simulink model "full_diffdrive_ctrl_sim_and_exp_with_arduino"  (R2020a)
settings: Solver=ode3  StartTime=0.0  StopTime=20  FixedStep=0.01  RelTol=1e-3  EnableMultiTasking=on
libraries: xpcobsoletelib x11, simulink x9, arduinolib x4, xpcutilitieslib x3, xpcrtudplib x2, slrtlib x1
(part 1 of 2)
settings Model: SILPILModeSetting=veronly  ExtModeTrigDuration=2  Creator=Boreth  LastModifiedBy=Boreth
settings DataIOCC: ReturnWorkspaceOutputs=off
settings OptimizationCC: EnhancedBackFolding=on  PassReuseOutputArgsAs=Individual arguments  MaxStackSize=64  OptimizeBlockOrder=speed  DifferentSizesBufferReuse=on  OptimizationCustomize=off  EfficientTunableParamExpr=on
settings DebuggingCC: InheritedTsInSrcMsg=none  ParameterTunabilityLossMsg=error  ArithmeticOperatorsInVariantConditions=warning
settings HardwareCC: ProdBitPerPointer=32  ProdBitPerSizeT=32  ProdBitPerPtrDiffT=32  ProdLargestAtomicInteger=Long  ProdLargestAtomicFloat=Double  ProdWordSize=32  ProdHWDeviceType=ARM Compatible->ARM Cortex
settings SFSimCC: MATLABDynamicMemAlloc=off  CustomCodeUndefinedFunction=UseInterfaceOnly
settings RTWCC: SystemTargetFile=ert.tlc  HardwareBoard=Arduino Due  TLCOptions=-aInlineSetEventsForThisBaseRateFcn=TLC_FALSE -aSuppressMultiTaskScheduler=TLC_FALSE -aRateBasedStepFcn=1  TemplateMakefile=ert_default_tmf  GenerateReport=on  Toolchain=Arduino ARM  BuildConfiguration=Faster Runs  IncludeHyperlinkInReport=on  LaunchReport=on  GenerateTraceInfo=on  GenerateTraceReport=on  GenerateTraceReportSl=on  GenerateTraceReportSf=on  GenerateTraceReportEml=on
settings CodeAppCC: ForceParamTrailComments=on  IgnoreCustomStorageClasses=off  OperatorAnnotations=on  SimulinkDataObjDesc=on  SFDataObjDesc=on  InsertBlockDesc=on
settings ERTTargetCC: SupportContinuousTime=on  SupportVariableSizeSignals=on  ExtModeStaticAllocSize=24576

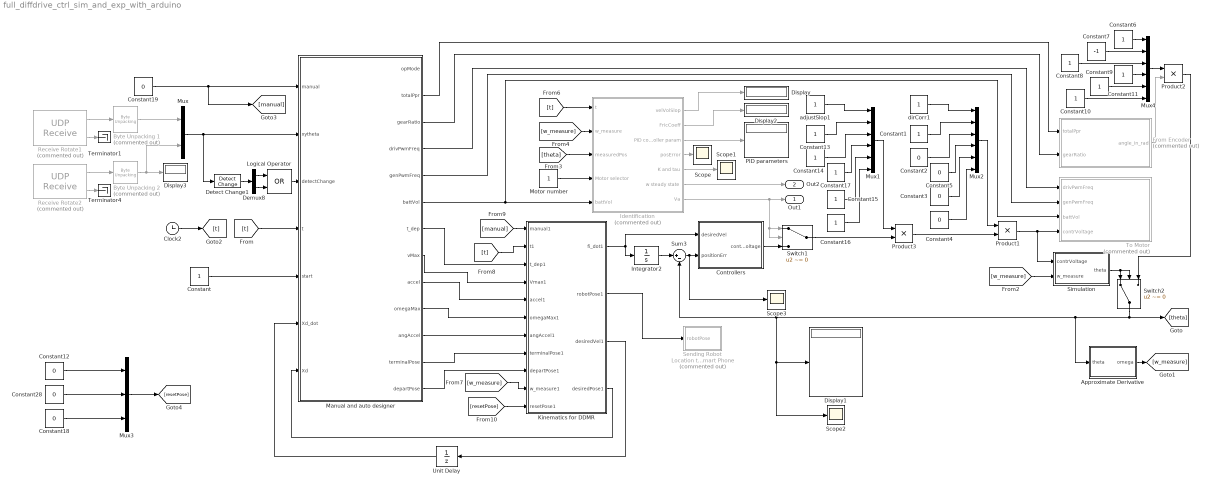
== system full_diffdrive_ctrl_sim_and_exp_with_arduino ==
  Approximate Derivative : Subsystem
  Byte Unpacking 1 : xpcutilitieslib/Byte Unpacking   Commented=on  MaskUnpackedDataTypes={'double'}  MaskUnpackedDataSizes={[1]}  MaskAlignment=1
      settings: SourceProductBaseCode=XP
  Byte Unpacking 2 : xpcutilitieslib/Byte Unpacking   Commented=on  MaskUnpackedDataTypes={'double'}  MaskUnpackedDataSizes={[1]}  MaskAlignment=1
      settings: SourceProductBaseCode=XP
  Clock2 : Clock
  Constant{,1,6,8..11,13..17} (12 alike) : Constant
  Constant{2..5,12,18..19,28} (8 alike) : Constant  Value=0
  Constant7 : Constant  Value=-1
  Controllers : Subsystem
  Demux8 : Demux  Outputs=2
  Detect Change1 : simulink/Logic and Bit Operations/Detect Change  vinit=0  OutDataTypeStr=boolean
  Display{,1..3} (4 alike) : Display
  From Encoder : Subsystem  Commented=on
  Identification : Subsystem  Commented=on
  Integrator2 : Integrator  InitialCondition=zeros(6,1)
  Kinematics for DDMR : Subsystem
  Logical Operator : Logic  Operator=OR  AllPortsSameDT=off  OutDataTypeStr=boolean
  Manual and auto designer : Stateflow chart  TreatAsAtomicUnit=on
  Motor number : Constant
  Mux : Mux  Inputs=2
  Mux1 : Mux  Inputs=6
  Mux2 : Mux  Inputs=6
  Mux3 : Mux  Inputs=3
  Mux4 : Mux  Inputs=6
  PID parameters : Display
  Product1 : Product
  Product2 : Product
  Product3 : Product
  Receive Rotate1 : xpcrtudplib/UDP Receive  Commented=on  ipAddressVal=Use host-target connection  localPort=2501  rcvWidth=8  rcvFmAny=off  fmAddress=192.168.88.233  rcvMulticast=off  multicastAddress={}  maxUDPQueue=8  sampleTime=-1
  Receive Rotate2 : xpcrtudplib/UDP Receive  Commented=on  ipAddressVal=Use host-target connection  localPort=2502  rcvWidth=8  rcvFmAny=off  fmAddress=192.168.88.233  rcvMulticast=off  multicastAddress={}  maxUDPQueue=8  sampleTime=-1
  Scope{,1..3} (4 alike) : Scope
  Sending Robot Location to Smart Phone : Subsystem  Commented=on
  Simulation : Subsystem
  Sum3 : Sum  Inputs=|+-
  Switch1 : Switch  Criteria=u2 ~= 0
  Switch2 : Switch  Criteria=u2 ~= 0
  Terminator1 : Terminator
  Terminator4 : Terminator
  To Motor : Subsystem  Commented=on
  Unit Delay : UnitDelay  InitialCondition=[0;0;0]  SampleTime=-1  HasFrameUpgradeWarning=on
  adjustSlop1 : Constant
  dirCorr1 : Constant
  Out1 : Outport
  Out2 : Outport  Port=2
  wires:
  [t] -> Manual and auto designer/4(t)
  Kinematics for DDMR/3(desiredVel1) -> Unit Delay/1
  Identification/5(K and tau) -> Scope1/1
  Kinematics for DDMR/2(robotPose1) -> Sending Robot Location to Smart Phone/1(robotPose)
  Manual and auto designer/12(terminalPose) -> Kinematics for DDMR/8(terminalPose1)
  Byte Unpacking 2/1 -> Mux/2, Display3/1
  Approximate Derivative/1(omega) -> [w_measure]
  Manual and auto designer/9(accel) -> Kinematics for DDMR/5(accel1)
  Demux8/2 -> Logical Operator/2
  Receive Rotate1/1 -> Byte Unpacking 1/1
  Manual and auto designer/6(battVol) -> To Motor/3(battVol), Identification/5(battVol)
  Manual and auto designer/13(departPose) -> Kinematics for DDMR/9(departPose1)
  [resetPose] -> Kinematics for DDMR/11(resetPose1)
  Mux/1 -> Detect Change1/1, Manual and auto designer/2(xytheta)
  Constant/1 -> Manual and auto designer/5(start)
  Demux8/1 -> Logical Operator/1
  Receive Rotate2/2 -> Terminator4/1
  Kinematics for DDMR/4(desiredPose1) -> Manual and auto designer/7(Xd)
  Manual and auto designer/8(vMax) -> Kinematics for DDMR/4(Vmax1)
  Identification/1(velVolSlop) -> Display/1
  Identification/4(posError) -> Scope/1
  Receive Rotate2/1 -> Byte Unpacking 2/1
  Byte Unpacking 1/1 -> Mux/1
  Product3/1 -> Product1/2
  Mux3/1 -> [resetPose]
  Manual and auto designer/7(t_dep) -> Kinematics for DDMR/3(t_dep1)
  [t] -> Kinematics for DDMR/2(t1)
  Manual and auto designer/10(omegaMax) -> Kinematics for DDMR/6(omegaMax1)
  Receive Rotate1/2 -> Terminator1/1
  Manual and auto designer/11(angAccel) -> Kinematics for DDMR/7(angAccel1)
  Unit Delay/1 -> Manual and auto designer/6(Xd_dot)
  Product1/1 -> Simulation/1(contrVoltage), To Motor/4(contrVoltage)
  Clock2/1 -> [t]
  Detect Change1/1 -> Demux8/1
  [w_measure] -> Simulation/2(w_measure)
  [manual] -> Kinematics for DDMR/1(manual1)
  Constant12/1 -> Mux3/1
  Constant19/1 -> [manual], Manual and auto designer/1(manual)
  Controllers/1(contrVoltage) -> Switch1/3
  Identification/3(PID controller param) -> PID parameters/1
  Constant10/1 -> Mux4/6
  Manual and auto designer/4(drivPwmFreq) -> To Motor/1(drivPwmFreq)
  [w_measure] -> Identification/2(w_measure)
  Kinematics for DDMR/1(fi_dot1) -> Integrator2/1, Controllers/1(desiredVel)
  Constant18/1 -> Mux3/3
  [theta] -> Identification/3(measuredPos)
  Motor number/1 -> Identification/4(Motor selector)
  Constant11/1 -> Mux4/4
  Integrator2/1 -> Sum3/1
  Identification/6(w steady state) -> Out2/1
  Switch1/1 -> Product3/2
  Simulation/1(theta) -> Switch2/2, Switch2/1
  Constant13/1 -> Mux1/2
  Manual and auto designer/2(totalPpr) -> From Encoder/1(totalPpr)
  Constant28/1 -> Mux3/2
  Constant14/1 -> Mux1/3
  From Encoder/1(angle_in_rad) -> Product2/2
  [w_measure] -> Kinematics for DDMR/10(w_measure1)
  Sum3/1 -> Scope3/1, Controllers/2(positionErr)
  adjustSlop1/1 -> Mux1/1
  Constant1/1 -> Mux2/2
  Identification/2(FricCoeff) -> Display2/1
  Identification/7(Va) -> Out1/1, Switch1/2, Switch1/1
  Mux1/1 -> Product3/1
  Constant17/1 -> Mux1/4
  Constant3/1 -> Mux2/5
  Manual and auto designer/5(genPwmFreq) -> To Motor/2(genPwmFreq)
  Constant16/1 -> Mux1/6
  Constant15/1 -> Mux1/5
  Manual and auto designer/3(gearRatio) -> From Encoder/2(gearRatio)
  Constant9/1 -> Mux4/5
  Mux4/1 -> Product2/1
  Constant8/1 -> Mux4/3
  Switch2/1 -> Approximate Derivative/1(theta), Sum3/2, Scope2/1, Display1/1, [theta]
  Mux2/1 -> Product1/1
  Constant5/1 -> Mux2/4
  dirCorr1/1 -> Mux2/1
  [t] -> Identification/1(t)
  Constant7/1 -> Mux4/2
  Constant6/1 -> Mux4/1
  Constant4/1 -> Mux2/6
  Logical Operator/1 -> Manual and auto designer/3(detectChange)
  Product2/1 -> Switch2/3
  Constant2/1 -> Mux2/3

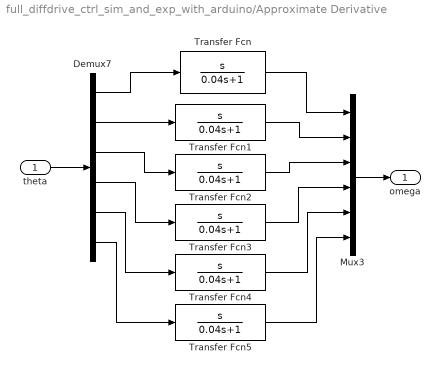
== system full_diffdrive_ctrl_sim_and_exp_with_arduino/Approximate Derivative ==
  theta : Inport
  Demux7 : Demux  Outputs=6
  Mux3 : Mux  Inputs=6
  Transfer Fcn{,1..5} (6 alike) : TransferFcn  Numerator=[1 0]  Denominator=[0.04 1]
  omega : Outport
  wires:
  Transfer Fcn1/1 -> Mux3/2
  Demux7/5 -> Transfer Fcn4/1
  Transfer Fcn3/1 -> Mux3/4
  Demux7/3 -> Transfer Fcn2/1
  Demux7/6 -> Transfer Fcn5/1
  Transfer Fcn2/1 -> Mux3/3
  Transfer Fcn/1 -> Mux3/1
  Transfer Fcn5/1 -> Mux3/6
  Demux7/4 -> Transfer Fcn3/1
  Mux3/1 -> omega/1
  Transfer Fcn4/1 -> Mux3/5
  Demux7/1 -> Transfer Fcn/1
  Demux7/2 -> Transfer Fcn1/1
  theta/1 -> Demux7/1

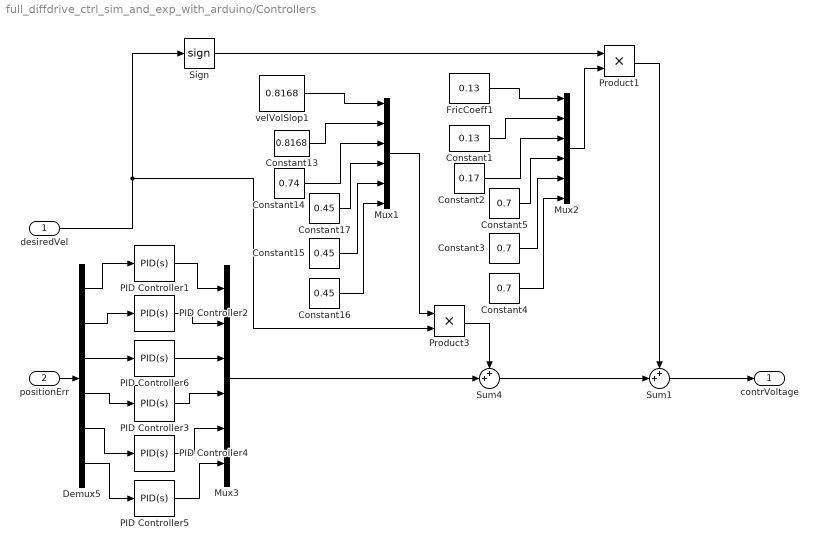
== system full_diffdrive_ctrl_sim_and_exp_with_arduino/Controllers ==
  desiredVel : Inport
  positionErr : Inport  Port=2
  Constant1 : Constant  Value=0.13
  Constant13 : Constant  Value=0.8168
  Constant14 : Constant  Value=0.74
  Constant15 : Constant  Value=0.45
  Constant16 : Constant  Value=0.45
  Constant17 : Constant  Value=0.45
  Constant2 : Constant  Value=0.17
  Constant3 : Constant  Value=0.7
  Constant4 : Constant  Value=0.7
  Constant5 : Constant  Value=0.7
  Demux5 : Demux  Outputs=6
  FricCoeff1 : Constant  Value=0.13
  Mux1 : Mux  Inputs=6
  Mux2 : Mux  Inputs=6
  Mux3 : Mux  Inputs=6
  "PID Controller1 " : simulink/Continuous/PID Controller  Controller=PID  Form=Parallel  TimeDomain=Continuous-time  UseExternalTs=off  SampleTime=-1  IntegratorMethod=Forward Euler  FilterMethod=Forward Euler  ControllerParametersSource=internal  P=13  I=0  D=1.522  UseFilter=on  N=50  TunerSelectOption=Transfer Function Based (PID Tuner App)  InitialConditionSource=internal  InitialConditionForIntegrator=0  InitialConditionForFilter=0  DifferentiatorICPrevScaledInput=0  ExternalReset=none  TrackingMode=off  Kt=1  LimitOutput=off  UpperSaturationLimit=inf  LowerSaturationLimit=-inf  LinearizeAsGain=on  AntiWindupMode=none  Kb=1  POutMin=[]  POutMax=[]  IOutMin=[]  IOutMax=[]  DOutMin=[]  DOutMax=[]  NOutMin=[]  NOutMax=[]  SumOutMin=[]  SumOutMax=[]  SaturationOutMin=[]  SaturationOutMax=[]  PParamMin=[]  PParamMax=[]  IParamMin=[]  IParamMax=[]  DParamMin=[]  DParamMax=[]  NParamMin=[]  NParamMax=[]  KbParamMin=[]  KbParamMax=[]  KtParamMin=[]  KtParamMax=[]  KbOutMin=[]  KbOutMax=[]  KtOutMin=[]  KtOutMax=[]  IntegratorOutMin=[]  IntegratorOutMax=[]  FilterOutMin=[]  FilterOutMax=[]  SumI1OutMin=[]  SumI1OutMax=[]  SumI2OutMin=[]  SumI2OutMax=[]  SumI3OutMin=[]  SumI3OutMax=[]  SumI4OutMin=[]  SumI4OutMax=[]  SumDOutMin=[]  SumDOutMax=[]  DifferentiatorOutMin=[]  DifferentiatorOutMax=[]  FilterDiffOutCoefMin=[]  FilterDiffOutCoefMax=[]  ReciprocalOutMin=[]  ReciprocalOutMax=[]  SumDenOutMin=[]  SumDenOutMax=[]  SumNumOutMin=[]  SumNumOutMax=[]  DivideOutMin=[]  DivideOutMax=[]  UdiffTsProdOutMin=[]  UdiffTsProdOutMax=[]  NTsProdOutMin=[]  NTsProdOutMax=[]  UintegralTsProdOutMin=[]  UintegralTsProdOutMax=[]  UngainTsProdOutMin=[]  UngainTsProdOutMax=[]  IntegratorContinuousStateAttributes=''  IntegratorStateMustResolveToSignalObject=off  IntegratorRTWStateStorageClass=Auto  FilterContinuousStateAttributes=''  FilterStateMustResolveToSignalObject=off  FilterRTWStateStorageClass=Auto  ParallelPVariant=InternalParameters  IdealPVariant=Disabled  IVariant=InternalParameters  DVariant=InternalParameters  IntegratorVariant=Continuous  SatVariant=Disabled  AWVariant=Passthrough  PCopyVariant=Disabled  TRVariant=Disabled  FdbkBlocksVariant=Forward  IdealPFdbkVariant=Disabled  SatFdbkVariant=Disabled  DerivativeFilterVariant=ContFilter  NVariant=InternalParameters  NCopyVariant=Disabled  FilterICVariant=InternalICsFilter  IntegratorICVariant=InternalICs  ExternalResetVariant=Disabled  TRSumVariant=Passthrough  SumFdbkVariant=Disabled  SumVariant=Sum_PID  TsampFilterVariant=InternalTs  TsampNgainVariant=Passthrough  TsampIntegralVariant=Passthrough
  PID Controller2 : simulink/Continuous/PID Controller  Controller=PID  Form=Parallel  TimeDomain=Continuous-time  UseExternalTs=off  SampleTime=-1  IntegratorMethod=Forward Euler  FilterMethod=Forward Euler  ControllerParametersSource=internal  P=13  I=0  D=1.522  UseFilter=on  N=100  TunerSelectOption=Transfer Function Based (PID Tuner App)  InitialConditionSource=internal  InitialConditionForIntegrator=0  InitialConditionForFilter=0  DifferentiatorICPrevScaledInput=0  ExternalReset=none  TrackingMode=off  Kt=1  LimitOutput=off  UpperSaturationLimit=inf  LowerSaturationLimit=-inf  LinearizeAsGain=on  AntiWindupMode=none  Kb=1  POutMin=[]  POutMax=[]  IOutMin=[]  IOutMax=[]  DOutMin=[]  DOutMax=[]  NOutMin=[]  NOutMax=[]  SumOutMin=[]  SumOutMax=[]  SaturationOutMin=[]  SaturationOutMax=[]  PParamMin=[]  PParamMax=[]  IParamMin=[]  IParamMax=[]  DParamMin=[]  DParamMax=[]  NParamMin=[]  NParamMax=[]  KbParamMin=[]  KbParamMax=[]  KtParamMin=[]  KtParamMax=[]  KbOutMin=[]  KbOutMax=[]  KtOutMin=[]  KtOutMax=[]  IntegratorOutMin=[]  IntegratorOutMax=[]  FilterOutMin=[]  FilterOutMax=[]  SumI1OutMin=[]  SumI1OutMax=[]  SumI2OutMin=[]  SumI2OutMax=[]  SumI3OutMin=[]  SumI3OutMax=[]  SumI4OutMin=[]  SumI4OutMax=[]  SumDOutMin=[]  SumDOutMax=[]  DifferentiatorOutMin=[]  DifferentiatorOutMax=[]  FilterDiffOutCoefMin=[]  FilterDiffOutCoefMax=[]  ReciprocalOutMin=[]  ReciprocalOutMax=[]  SumDenOutMin=[]  SumDenOutMax=[]  SumNumOutMin=[]  SumNumOutMax=[]  DivideOutMin=[]  DivideOutMax=[]  UdiffTsProdOutMin=[]  UdiffTsProdOutMax=[]  NTsProdOutMin=[]  NTsProdOutMax=[]  UintegralTsProdOutMin=[]  UintegralTsProdOutMax=[]  UngainTsProdOutMin=[]  UngainTsProdOutMax=[]  IntegratorContinuousStateAttributes=''  IntegratorStateMustResolveToSignalObject=off  IntegratorRTWStateStorageClass=Auto  FilterContinuousStateAttributes=''  FilterStateMustResolveToSignalObject=off  FilterRTWStateStorageClass=Auto  ParallelPVariant=InternalParameters  IdealPVariant=Disabled  IVariant=InternalParameters  DVariant=InternalParameters  IntegratorVariant=Continuous  SatVariant=Disabled  AWVariant=Passthrough  PCopyVariant=Disabled  TRVariant=Disabled  FdbkBlocksVariant=Forward  IdealPFdbkVariant=Disabled  SatFdbkVariant=Disabled  DerivativeFilterVariant=ContFilter  NVariant=InternalParameters  NCopyVariant=Disabled  FilterICVariant=InternalICsFilter  IntegratorICVariant=InternalICs  ExternalResetVariant=Disabled  TRSumVariant=Passthrough  SumFdbkVariant=Disabled  SumVariant=Sum_PID  TsampFilterVariant=InternalTs  TsampNgainVariant=Passthrough  TsampIntegralVariant=Passthrough
  PID Controller3 : simulink/Continuous/PID Controller  Controller=PID  Form=Parallel  TimeDomain=Continuous-time  UseExternalTs=off  SampleTime=-1  IntegratorMethod=Forward Euler  FilterMethod=Forward Euler  ControllerParametersSource=internal  P=10  I=0  D=3  UseFilter=on  N=100  TunerSelectOption=Transfer Function Based (PID Tuner App)  InitialConditionSource=internal  InitialConditionForIntegrator=0  InitialConditionForFilter=0  DifferentiatorICPrevScaledInput=0  ExternalReset=none  TrackingMode=off  Kt=1  LimitOutput=off  UpperSaturationLimit=inf  LowerSaturationLimit=-inf  LinearizeAsGain=on  AntiWindupMode=none  Kb=1  POutMin=[]  POutMax=[]  IOutMin=[]  IOutMax=[]  DOutMin=[]  DOutMax=[]  NOutMin=[]  NOutMax=[]  SumOutMin=[]  SumOutMax=[]  SaturationOutMin=[]  SaturationOutMax=[]  PParamMin=[]  PParamMax=[]  IParamMin=[]  IParamMax=[]  DParamMin=[]  DParamMax=[]  NParamMin=[]  NParamMax=[]  KbParamMin=[]  KbParamMax=[]  KtParamMin=[]  KtParamMax=[]  KbOutMin=[]  KbOutMax=[]  KtOutMin=[]  KtOutMax=[]  IntegratorOutMin=[]  IntegratorOutMax=[]  FilterOutMin=[]  FilterOutMax=[]  SumI1OutMin=[]  SumI1OutMax=[]  SumI2OutMin=[]  SumI2OutMax=[]  SumI3OutMin=[]  SumI3OutMax=[]  SumI4OutMin=[]  SumI4OutMax=[]  SumDOutMin=[]  SumDOutMax=[]  DifferentiatorOutMin=[]  DifferentiatorOutMax=[]  FilterDiffOutCoefMin=[]  FilterDiffOutCoefMax=[]  ReciprocalOutMin=[]  ReciprocalOutMax=[]  SumDenOutMin=[]  SumDenOutMax=[]  SumNumOutMin=[]  SumNumOutMax=[]  DivideOutMin=[]  DivideOutMax=[]  UdiffTsProdOutMin=[]  UdiffTsProdOutMax=[]  NTsProdOutMin=[]  NTsProdOutMax=[]  UintegralTsProdOutMin=[]  UintegralTsProdOutMax=[]  UngainTsProdOutMin=[]  UngainTsProdOutMax=[]  IntegratorContinuousStateAttributes=''  IntegratorStateMustResolveToSignalObject=off  IntegratorRTWStateStorageClass=Auto  FilterContinuousStateAttributes=''  FilterStateMustResolveToSignalObject=off  FilterRTWStateStorageClass=Auto  ParallelPVariant=InternalParameters  IdealPVariant=Disabled  IVariant=InternalParameters  DVariant=InternalParameters  IntegratorVariant=Continuous  SatVariant=Disabled  AWVariant=Passthrough  PCopyVariant=Disabled  TRVariant=Disabled  FdbkBlocksVariant=Forward  IdealPFdbkVariant=Disabled  SatFdbkVariant=Disabled  DerivativeFilterVariant=ContFilter  NVariant=InternalParameters  NCopyVariant=Disabled  FilterICVariant=InternalICsFilter  IntegratorICVariant=InternalICs  ExternalResetVariant=Disabled  TRSumVariant=Passthrough  SumFdbkVariant=Disabled  SumVariant=Sum_PID  TsampFilterVariant=InternalTs  TsampNgainVariant=Passthrough  TsampIntegralVariant=Passthrough
  PID Controller4 : simulink/Continuous/PID Controller  Controller=PID  Form=Parallel  TimeDomain=Continuous-time  UseExternalTs=off  SampleTime=-1  IntegratorMethod=Forward Euler  FilterMethod=Forward Euler  ControllerParametersSource=internal  P=10  I=0  D=3  UseFilter=on  N=100  TunerSelectOption=Transfer Function Based (PID Tuner App)  InitialConditionSource=internal  InitialConditionForIntegrator=0  InitialConditionForFilter=0  DifferentiatorICPrevScaledInput=0  ExternalReset=none  TrackingMode=off  Kt=1  LimitOutput=off  UpperSaturationLimit=inf  LowerSaturationLimit=-inf  LinearizeAsGain=on  AntiWindupMode=none  Kb=1  POutMin=[]  POutMax=[]  IOutMin=[]  IOutMax=[]  DOutMin=[]  DOutMax=[]  NOutMin=[]  NOutMax=[]  SumOutMin=[]  SumOutMax=[]  SaturationOutMin=[]  SaturationOutMax=[]  PParamMin=[]  PParamMax=[]  IParamMin=[]  IParamMax=[]  DParamMin=[]  DParamMax=[]  NParamMin=[]  NParamMax=[]  KbParamMin=[]  KbParamMax=[]  KtParamMin=[]  KtParamMax=[]  KbOutMin=[]  KbOutMax=[]  KtOutMin=[]  KtOutMax=[]  IntegratorOutMin=[]  IntegratorOutMax=[]  FilterOutMin=[]  FilterOutMax=[]  SumI1OutMin=[]  SumI1OutMax=[]  SumI2OutMin=[]  SumI2OutMax=[]  SumI3OutMin=[]  SumI3OutMax=[]  SumI4OutMin=[]  SumI4OutMax=[]  SumDOutMin=[]  SumDOutMax=[]  DifferentiatorOutMin=[]  DifferentiatorOutMax=[]  FilterDiffOutCoefMin=[]  FilterDiffOutCoefMax=[]  ReciprocalOutMin=[]  ReciprocalOutMax=[]  SumDenOutMin=[]  SumDenOutMax=[]  SumNumOutMin=[]  SumNumOutMax=[]  DivideOutMin=[]  DivideOutMax=[]  UdiffTsProdOutMin=[]  UdiffTsProdOutMax=[]  NTsProdOutMin=[]  NTsProdOutMax=[]  UintegralTsProdOutMin=[]  UintegralTsProdOutMax=[]  UngainTsProdOutMin=[]  UngainTsProdOutMax=[]  IntegratorContinuousStateAttributes=''  IntegratorStateMustResolveToSignalObject=off  IntegratorRTWStateStorageClass=Auto  FilterContinuousStateAttributes=''  FilterStateMustResolveToSignalObject=off  FilterRTWStateStorageClass=Auto  ParallelPVariant=InternalParameters  IdealPVariant=Disabled  IVariant=InternalParameters  DVariant=InternalParameters  IntegratorVariant=Continuous  SatVariant=Disabled  AWVariant=Passthrough  PCopyVariant=Disabled  TRVariant=Disabled  FdbkBlocksVariant=Forward  IdealPFdbkVariant=Disabled  SatFdbkVariant=Disabled  DerivativeFilterVariant=ContFilter  NVariant=InternalParameters  NCopyVariant=Disabled  FilterICVariant=InternalICsFilter  IntegratorICVariant=InternalICs  ExternalResetVariant=Disabled  TRSumVariant=Passthrough  SumFdbkVariant=Disabled  SumVariant=Sum_PID  TsampFilterVariant=InternalTs  TsampNgainVariant=Passthrough  TsampIntegralVariant=Passthrough
  PID Controller5 : simulink/Continuous/PID Controller  Controller=PID  Form=Parallel  TimeDomain=Continuous-time  UseExternalTs=off  SampleTime=-1  IntegratorMethod=Forward Euler  FilterMethod=Forward Euler  ControllerParametersSource=internal  P=10  I=0  D=3  UseFilter=on  N=100  TunerSelectOption=Transfer Function Based (PID Tuner App)  InitialConditionSource=internal  InitialConditionForIntegrator=0  InitialConditionForFilter=0  DifferentiatorICPrevScaledInput=0  ExternalReset=none  TrackingMode=off  Kt=1  LimitOutput=off  UpperSaturationLimit=inf  LowerSaturationLimit=-inf  LinearizeAsGain=on  AntiWindupMode=none  Kb=1  POutMin=[]  POutMax=[]  IOutMin=[]  IOutMax=[]  DOutMin=[]  DOutMax=[]  NOutMin=[]  NOutMax=[]  SumOutMin=[]  SumOutMax=[]  SaturationOutMin=[]  SaturationOutMax=[]  PParamMin=[]  PParamMax=[]  IParamMin=[]  IParamMax=[]  DParamMin=[]  DParamMax=[]  NParamMin=[]  NParamMax=[]  KbParamMin=[]  KbParamMax=[]  KtParamMin=[]  KtParamMax=[]  KbOutMin=[]  KbOutMax=[]  KtOutMin=[]  KtOutMax=[]  IntegratorOutMin=[]  IntegratorOutMax=[]  FilterOutMin=[]  FilterOutMax=[]  SumI1OutMin=[]  SumI1OutMax=[]  SumI2OutMin=[]  SumI2OutMax=[]  SumI3OutMin=[]  SumI3OutMax=[]  SumI4OutMin=[]  SumI4OutMax=[]  SumDOutMin=[]  SumDOutMax=[]  DifferentiatorOutMin=[]  DifferentiatorOutMax=[]  FilterDiffOutCoefMin=[]  FilterDiffOutCoefMax=[]  ReciprocalOutMin=[]  ReciprocalOutMax=[]  SumDenOutMin=[]  SumDenOutMax=[]  SumNumOutMin=[]  SumNumOutMax=[]  DivideOutMin=[]  DivideOutMax=[]  UdiffTsProdOutMin=[]  UdiffTsProdOutMax=[]  NTsProdOutMin=[]  NTsProdOutMax=[]  UintegralTsProdOutMin=[]  UintegralTsProdOutMax=[]  UngainTsProdOutMin=[]  UngainTsProdOutMax=[]  IntegratorContinuousStateAttributes=''  IntegratorStateMustResolveToSignalObject=off  IntegratorRTWStateStorageClass=Auto  FilterContinuousStateAttributes=''  FilterStateMustResolveToSignalObject=off  FilterRTWStateStorageClass=Auto  ParallelPVariant=InternalParameters  IdealPVariant=Disabled  IVariant=InternalParameters  DVariant=InternalParameters  IntegratorVariant=Continuous  SatVariant=Disabled  AWVariant=Passthrough  PCopyVariant=Disabled  TRVariant=Disabled  FdbkBlocksVariant=Forward  IdealPFdbkVariant=Disabled  SatFdbkVariant=Disabled  DerivativeFilterVariant=ContFilter  NVariant=InternalParameters  NCopyVariant=Disabled  FilterICVariant=InternalICsFilter  IntegratorICVariant=InternalICs  ExternalResetVariant=Disabled  TRSumVariant=Passthrough  SumFdbkVariant=Disabled  SumVariant=Sum_PID  TsampFilterVariant=InternalTs  TsampNgainVariant=Passthrough  TsampIntegralVariant=Passthrough
  PID Controller6 : simulink/Continuous/PID Controller  Controller=PID  Form=Parallel  TimeDomain=Continuous-time  UseExternalTs=off  SampleTime=-1  IntegratorMethod=Forward Euler  FilterMethod=Forward Euler  ControllerParametersSource=internal  P=45/0.74  I=0  D=2.59/0.74  UseFilter=on  N=100  TunerSelectOption=Transfer Function Based (PID Tuner App)  InitialConditionSource=internal  InitialConditionForIntegrator=0  InitialConditionForFilter=0  DifferentiatorICPrevScaledInput=0  ExternalReset=none  TrackingMode=off  Kt=1  LimitOutput=off  UpperSaturationLimit=inf  LowerSaturationLimit=-inf  LinearizeAsGain=on  AntiWindupMode=none  Kb=1  POutMin=[]  POutMax=[]  IOutMin=[]  IOutMax=[]  DOutMin=[]  DOutMax=[]  NOutMin=[]  NOutMax=[]  SumOutMin=[]  SumOutMax=[]  SaturationOutMin=[]  SaturationOutMax=[]  PParamMin=[]  PParamMax=[]  IParamMin=[]  IParamMax=[]  DParamMin=[]  DParamMax=[]  NParamMin=[]  NParamMax=[]  KbParamMin=[]  KbParamMax=[]  KtParamMin=[]  KtParamMax=[]  KbOutMin=[]  KbOutMax=[]  KtOutMin=[]  KtOutMax=[]  IntegratorOutMin=[]  IntegratorOutMax=[]  FilterOutMin=[]  FilterOutMax=[]  SumI1OutMin=[]  SumI1OutMax=[]  SumI2OutMin=[]  SumI2OutMax=[]  SumI3OutMin=[]  SumI3OutMax=[]  SumI4OutMin=[]  SumI4OutMax=[]  SumDOutMin=[]  SumDOutMax=[]  DifferentiatorOutMin=[]  DifferentiatorOutMax=[]  FilterDiffOutCoefMin=[]  FilterDiffOutCoefMax=[]  ReciprocalOutMin=[]  ReciprocalOutMax=[]  SumDenOutMin=[]  SumDenOutMax=[]  SumNumOutMin=[]  SumNumOutMax=[]  DivideOutMin=[]  DivideOutMax=[]  UdiffTsProdOutMin=[]  UdiffTsProdOutMax=[]  NTsProdOutMin=[]  NTsProdOutMax=[]  UintegralTsProdOutMin=[]  UintegralTsProdOutMax=[]  UngainTsProdOutMin=[]  UngainTsProdOutMax=[]  IntegratorContinuousStateAttributes=''  IntegratorStateMustResolveToSignalObject=off  IntegratorRTWStateStorageClass=Auto  FilterContinuousStateAttributes=''  FilterStateMustResolveToSignalObject=off  FilterRTWStateStorageClass=Auto  ParallelPVariant=InternalParameters  IdealPVariant=Disabled  IVariant=InternalParameters  DVariant=InternalParameters  IntegratorVariant=Continuous  SatVariant=Disabled  AWVariant=Passthrough  PCopyVariant=Disabled  TRVariant=Disabled  FdbkBlocksVariant=Forward  IdealPFdbkVariant=Disabled  SatFdbkVariant=Disabled  DerivativeFilterVariant=ContFilter  NVariant=InternalParameters  NCopyVariant=Disabled  FilterICVariant=InternalICsFilter  IntegratorICVariant=InternalICs  ExternalResetVariant=Disabled  TRSumVariant=Passthrough  SumFdbkVariant=Disabled  SumVariant=Sum_PID  TsampFilterVariant=InternalTs  TsampNgainVariant=Passthrough  TsampIntegralVariant=Passthrough
  Product1 : Product
  Product3 : Product
  Sign : Signum
  Sum1 : Sum  Inputs=++|
  Sum4 : Sum  Inputs=++|
  velVolSlop1 : Constant  Value=0.8168
  contrVoltage : Outport
  wires:
  PID Controller2/1 -> Mux3/2
  Demux5/3 -> PID Controller6/1
  Demux5/1 -> "PID Controller1 "/1
  PID Controller6/1 -> Mux3/3
  "PID Controller1 "/1 -> Mux3/1
  positionErr/1 -> Demux5/1
  Demux5/2 -> PID Controller2/1
  Demux5/4 -> PID Controller3/1
  Demux5/5 -> PID Controller4/1
  Demux5/6 -> PID Controller5/1
  PID Controller3/1 -> Mux3/4
  PID Controller4/1 -> Mux3/5
  PID Controller5/1 -> Mux3/6
  Constant16/1 -> Mux1/6
  Constant15/1 -> Mux1/5
  Constant14/1 -> Mux1/3
  Constant13/1 -> Mux1/2
  velVolSlop1/1 -> Mux1/1
  Mux1/1 -> Product3/1
  Constant17/1 -> Mux1/4
  Sum1/1 -> contrVoltage/1
  Mux3/1 -> Sum4/2
  desiredVel/1 -> Sign/1, Product3/2
  Sum4/1 -> Sum1/2
  Constant2/1 -> Mux2/3
  Constant5/1 -> Mux2/4
  FricCoeff1/1 -> Mux2/1
  Constant4/1 -> Mux2/6
  Constant3/1 -> Mux2/5
  Constant1/1 -> Mux2/2
  Sign/1 -> Product1/1
  Mux2/1 -> Product1/2
  Product1/1 -> Sum1/1
  Product3/1 -> Sum4/1

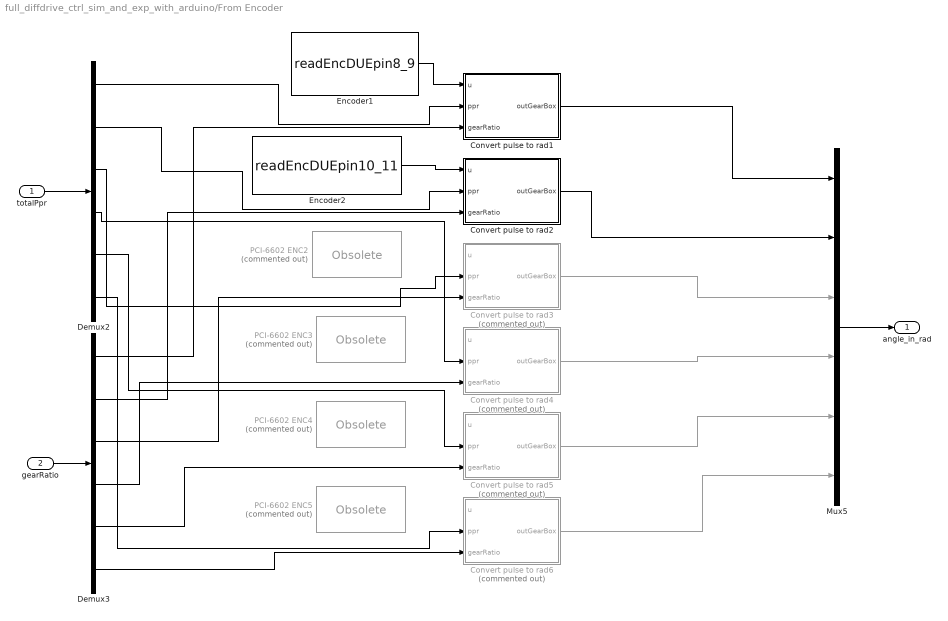
== system full_diffdrive_ctrl_sim_and_exp_with_arduino/From Encoder ==
  totalPpr : Inport
  gearRatio : Inport  Port=2
  Convert pulse to rad1 : MATLAB Function  TreatAsAtomicUnit=on
  Convert pulse to rad2 : MATLAB Function  TreatAsAtomicUnit=on
  Convert pulse to rad3 : MATLAB Function  Commented=on  TreatAsAtomicUnit=on
  Convert pulse to rad4 : MATLAB Function  Commented=on  TreatAsAtomicUnit=on
  Convert pulse to rad5 : MATLAB Function  Commented=on  TreatAsAtomicUnit=on
  Convert pulse to rad6 : MATLAB Function  Commented=on  TreatAsAtomicUnit=on
  Demux2 : Demux  Outputs=6
  Demux3 : Demux  Outputs=6
  Encoder1 : S-Function  InitFcn=try, set_param(gcb,'FunctionName','readEncDUEpin8_9'), end  FunctionName=readEncDUEpin8_9  SFunctionModules=readEncDUEpin8_9_wrapper  SFunctionDeploymentMode=off  EnableBusSupport=off  mask(S-Function Builder){}
      mask help: Simulink:masks:SFunctionBuilder_MD
      mask init:
      | val = [[.9  0.75 0.75 1 1 .9 .9 1]',[1 1 0.75 0.75 .9 .9 1 .9]'];try , sys = get_param(gcb,'SfunBuilderFcnName');if isempty(sys), sys = get_param(gcb,'FunctionName'); end,catch, sys = get_param(gcb,'FunctionName'); end
      settings: CopyFcn=set_param(gcbh,'LinkStatus','none')  PreSaveFcn=try, set_param(gcb,'FunctionName','readEncDUEpin8_9'), end  OpenFcn=sfunctionwizard(gcbh)
      mask Display: plot(val(:,1),val(:,2)),disp(sys), port_label('output',1,'count')
  Encoder2 : S-Function  InitFcn=try, set_param(gcb,'FunctionName','readEncDUEpin10_11'), end  FunctionName=readEncDUEpin10_11  SFunctionModules=readEncDUEpin10_11_wrapper  SFunctionDeploymentMode=off  EnableBusSupport=off  mask(S-Function Builder){}
      mask help: Simulink:masks:SFunctionBuilder_MD
      mask init: same as full_diffdrive_ctrl_sim_and_exp_with_arduino/From Encoder/Encoder1
      settings: CopyFcn=set_param(gcbh,'LinkStatus','none')  PreSaveFcn=try, set_param(gcb,'FunctionName','readEncDUEpin10_11'), end  OpenFcn=sfunctionwizard(gcbh)
      mask Display: plot(val(:,1),val(:,2)),disp(sys), port_label('output',1,'countt')
  Mux5 : Mux  Inputs=6
  PCI-6602 ENC{2..5} (4 alike) : xpcobsoletelib/Obsolete  Commented=on
      settings: SourceProductBaseCode=XP
  angle_in_rad : Outport
  wires:
  Demux3/5 -> Convert pulse to rad5/3(gearRatio)
  Demux3/6 -> Convert pulse to rad6/3(gearRatio)
  Demux3/1 -> Convert pulse to rad1/3(gearRatio)
  Convert pulse to rad3/1(outGearBox) -> Mux5/3
  Convert pulse to rad5/1(outGearBox) -> Mux5/5
  Mux5/1 -> angle_in_rad/1
  Demux2/2 -> Convert pulse to rad2/2(ppr)
  gearRatio/1 -> Demux3/1
  ? -> Convert pulse to rad5/1(u)
  Demux2/5 -> Convert pulse to rad5/2(ppr)
  ? -> Convert pulse to rad4/1(u)
  Demux2/6 -> Convert pulse to rad6/2(ppr)
  Demux2/3 -> Convert pulse to rad3/2(ppr)
  Demux3/3 -> Convert pulse to rad3/3(gearRatio)
  Encoder2/1 -> Convert pulse to rad2/1(u)
  Demux2/4 -> Convert pulse to rad4/2(ppr)
  Demux2/1 -> Convert pulse to rad1/2(ppr)
  Convert pulse to rad6/1(outGearBox) -> Mux5/6
  Demux3/4 -> Convert pulse to rad4/3(gearRatio)
  Convert pulse to rad1/1(outGearBox) -> Mux5/1
  ? -> Convert pulse to rad3/1(u)
  Convert pulse to rad4/1(outGearBox) -> Mux5/4
  Demux3/2 -> Convert pulse to rad2/3(gearRatio)
  Convert pulse to rad2/1(outGearBox) -> Mux5/2
  totalPpr/1 -> Demux2/1
  ? -> Convert pulse to rad6/1(u)
  Encoder1/1 -> Convert pulse to rad1/1(u)

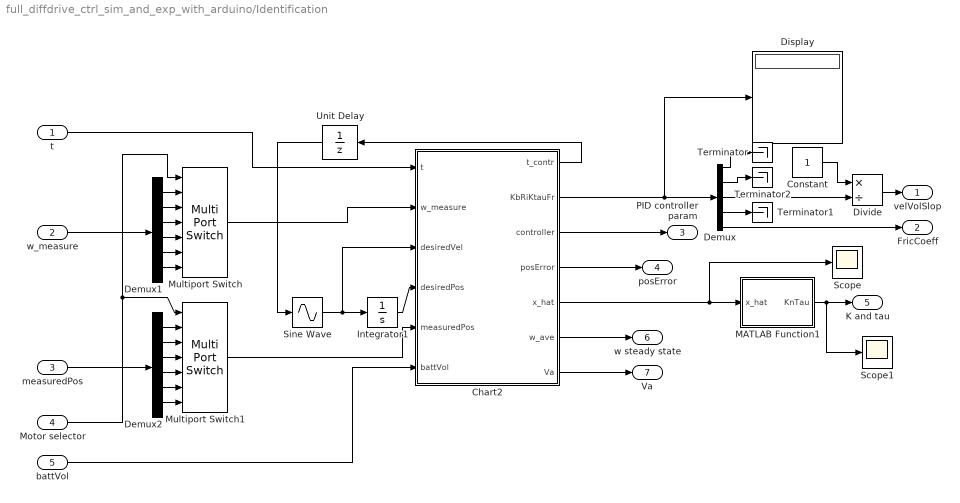
== system full_diffdrive_ctrl_sim_and_exp_with_arduino/Identification ==
  t : Inport
  w_measure : Inport  Port=2
  measuredPos : Inport  Port=3
  Motor selector : Inport  Port=4
  battVol : Inport  Port=5
  Chart2 : Stateflow chart  TreatAsAtomicUnit=on
  Constant : Constant
  Demux : Demux  Outputs=5
  Demux1 : Demux  Outputs=6
  Demux2 : Demux  Outputs=6
  Display : Display
  Divide : Product  Inputs=*/
  Integrator1 : Integrator
  MATLAB Function1 : MATLAB Function  TreatAsAtomicUnit=on
  Multiport Switch : MultiPortSwitch  Inputs=6
  Multiport Switch1 : MultiPortSwitch  Inputs=6
  Scope : Scope
  Scope1 : Scope
  Sine Wave : Sin  TimeSource=Use external signal  Amplitude=pi  SampleTime=0
  Terminator : Terminator
  Terminator1 : Terminator
  Terminator2 : Terminator
  Unit Delay : UnitDelay  SampleTime=-1  HasFrameUpgradeWarning=on
  velVolSlop : Outport
  FricCoeff : Outport  Port=2
  PID controller param : Outport  Port=3
  posError : Outport  Port=4
  K and tau : Outport  Port=5
  w steady state : Outport  Port=6
  Va : Outport  Port=7
  wires:
  Sine Wave/1 -> Chart2/3(desiredVel), Integrator1/1
  Chart2/5(x_hat) -> Scope/1, MATLAB Function1/1(x_hat)
  Multiport Switch/1 -> Chart2/2(w_measure)
  Chart2/7(Va) -> Va/1
  Chart2/1(t_contr) -> Unit Delay/1
  Integrator1/1 -> Chart2/4(desiredPos)
  Unit Delay/1 -> Sine Wave/1
  Chart2/4(posError) -> posError/1
  MATLAB Function1/1(KnTau) -> Scope1/1, K and tau/1
  Multiport Switch1/1 -> Chart2/5(measuredPos)
  t/1 -> Chart2/1(t)
  Chart2/2(KbRiKtauFr) -> Display/1, Demux/1
  Chart2/3(controller) -> PID controller param/1
  Chart2/6(w_ave) -> w steady state/1
  Demux/3 -> Divide/2
  Divide/1 -> velVolSlop/1
  Constant/1 -> Divide/1
  Demux/1 -> Terminator/1
  Demux/4 -> Terminator1/1
  Demux/2 -> Terminator2/1
  Demux1/1 -> Multiport Switch/2
  Demux1/2 -> Multiport Switch/3
  Demux1/3 -> Multiport Switch/4
  Demux1/4 -> Multiport Switch/5
  Demux1/5 -> Multiport Switch/6
  Demux1/6 -> Multiport Switch/7
  Demux2/1 -> Multiport Switch1/2
  Demux2/2 -> Multiport Switch1/3
  Demux2/3 -> Multiport Switch1/4
  Demux2/4 -> Multiport Switch1/5
  Demux2/5 -> Multiport Switch1/6
  Demux2/6 -> Multiport Switch1/7
  measuredPos/1 -> Demux2/1
  w_measure/1 -> Demux1/1
  Motor selector/1 -> Multiport Switch1/1, Multiport Switch/1
  Demux/5 -> FricCoeff/1
  battVol/1 -> Chart2/6(battVol)

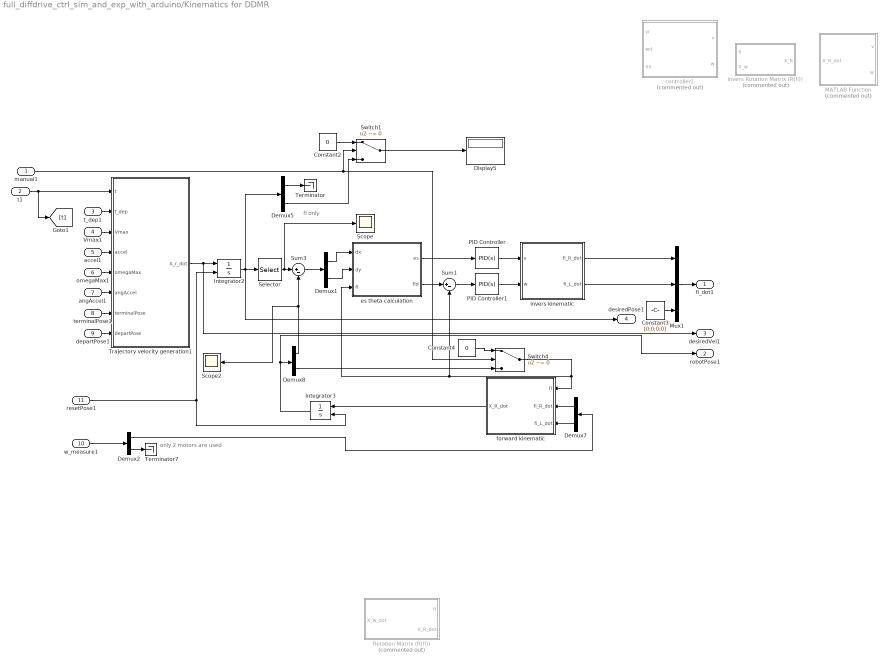
== system full_diffdrive_ctrl_sim_and_exp_with_arduino/Kinematics for DDMR ==
  note: fi only
  note: only 2 motors are used
  manual1 : Inport
  t1 : Inport  Port=2
  t_dep1 : Inport  Port=3
  Vmax1 : Inport  Port=4
  accel1 : Inport  Port=5
  omegaMax1 : Inport  Port=6
  angAccel1 : Inport  Port=7
  terminalPose1 : Inport  Port=8
  departPose1 : Inport  Port=9
  w_measure1 : Inport  Port=10
  resetPose1 : Inport  Port=11
  Constant2 : Constant  Value=0
  Constant3 : Constant  Value=[0;0;0;0]
  Constant4 : Constant  Value=0
  Demux1 : Demux  Outputs=2
  Demux2 : Demux  Outputs=[2,4]
  Demux5 : Demux  Outputs=[2 1]
  Demux7 : Demux  Outputs=2
  Demux8 : Demux  Outputs=[2 1]
  Display5 : Display
  Integrator2 : Integrator  ExternalReset=either  InitialCondition=[0;0;0]
  Integrator3 : Integrator  ExternalReset=either  InitialCondition=[0;0;0]
  MATLAB Function : MATLAB Function  Commented=on  TreatAsAtomicUnit=on
  Mux1 : Mux  Inputs=[1,1,4]
  PID Controller : simulink/Continuous/PID Controller  Controller=PID  Form=Parallel  TimeDomain=Continuous-time  UseExternalTs=off  SampleTime=-1  IntegratorMethod=Forward Euler  FilterMethod=Forward Euler  ControllerParametersSource=internal  P=1  I=0  D=0.01  UseFilter=on  N=100  TunerSelectOption=Transfer Function Based (PID Tuner App)  InitialConditionSource=internal  InitialConditionForIntegrator=0  InitialConditionForFilter=0  DifferentiatorICPrevScaledInput=0  ExternalReset=none  TrackingMode=off  Kt=1  LimitOutput=off  UpperSaturationLimit=inf  LowerSaturationLimit=-inf  LinearizeAsGain=on  AntiWindupMode=none  Kb=1  POutMin=[]  POutMax=[]  IOutMin=[]  IOutMax=[]  DOutMin=[]  DOutMax=[]  NOutMin=[]  NOutMax=[]  SumOutMin=[]  SumOutMax=[]  SaturationOutMin=[]  SaturationOutMax=[]  PParamMin=[]  PParamMax=[]  IParamMin=[]  IParamMax=[]  DParamMin=[]  DParamMax=[]  NParamMin=[]  NParamMax=[]  KbParamMin=[]  KbParamMax=[]  KtParamMin=[]  KtParamMax=[]  KbOutMin=[]  KbOutMax=[]  KtOutMin=[]  KtOutMax=[]  IntegratorOutMin=[]  IntegratorOutMax=[]  FilterOutMin=[]  FilterOutMax=[]  SumI1OutMin=[]  SumI1OutMax=[]  SumI2OutMin=[]  SumI2OutMax=[]  SumI3OutMin=[]  SumI3OutMax=[]  SumI4OutMin=[]  SumI4OutMax=[]  SumDOutMin=[]  SumDOutMax=[]  DifferentiatorOutMin=[]  DifferentiatorOutMax=[]  FilterDiffOutCoefMin=[]  FilterDiffOutCoefMax=[]  ReciprocalOutMin=[]  ReciprocalOutMax=[]  SumDenOutMin=[]  SumDenOutMax=[]  SumNumOutMin=[]  SumNumOutMax=[]  DivideOutMin=[]  DivideOutMax=[]  UdiffTsProdOutMin=[]  UdiffTsProdOutMax=[]  NTsProdOutMin=[]  NTsProdOutMax=[]  UintegralTsProdOutMin=[]  UintegralTsProdOutMax=[]  UngainTsProdOutMin=[]  UngainTsProdOutMax=[]  IntegratorContinuousStateAttributes=''  IntegratorStateMustResolveToSignalObject=off  IntegratorRTWStateStorageClass=Auto  FilterContinuousStateAttributes=''  FilterStateMustResolveToSignalObject=off  FilterRTWStateStorageClass=Auto  ParallelPVariant=InternalParameters  IdealPVariant=Disabled  IVariant=InternalParameters  DVariant=InternalParameters  IntegratorVariant=Continuous  SatVariant=Disabled  AWVariant=Passthrough  PCopyVariant=Disabled  TRVariant=Disabled  FdbkBlocksVariant=Forward  IdealPFdbkVariant=Disabled  SatFdbkVariant=Disabled  DerivativeFilterVariant=ContFilter  NVariant=InternalParameters  NCopyVariant=Disabled  FilterICVariant=InternalICsFilter  IntegratorICVariant=InternalICs  ExternalResetVariant=Disabled  TRSumVariant=Passthrough  SumFdbkVariant=Disabled  SumVariant=Sum_PID  TsampFilterVariant=InternalTs  TsampNgainVariant=Passthrough  TsampIntegralVariant=Passthrough
  PID Controller1 : simulink/Continuous/PID Controller  Controller=PID  Form=Parallel  TimeDomain=Continuous-time  UseExternalTs=off  SampleTime=-1  IntegratorMethod=Forward Euler  FilterMethod=Forward Euler  ControllerParametersSource=internal  P=1  I=0  D=0.01  UseFilter=on  N=100  TunerSelectOption=Transfer Function Based (PID Tuner App)  InitialConditionSource=internal  InitialConditionForIntegrator=0  InitialConditionForFilter=0  DifferentiatorICPrevScaledInput=0  ExternalReset=none  TrackingMode=off  Kt=1  LimitOutput=off  UpperSaturationLimit=inf  LowerSaturationLimit=-inf  LinearizeAsGain=on  AntiWindupMode=none  Kb=1  POutMin=[]  POutMax=[]  IOutMin=[]  IOutMax=[]  DOutMin=[]  DOutMax=[]  NOutMin=[]  NOutMax=[]  SumOutMin=[]  SumOutMax=[]  SaturationOutMin=[]  SaturationOutMax=[]  PParamMin=[]  PParamMax=[]  IParamMin=[]  IParamMax=[]  DParamMin=[]  DParamMax=[]  NParamMin=[]  NParamMax=[]  KbParamMin=[]  KbParamMax=[]  KtParamMin=[]  KtParamMax=[]  KbOutMin=[]  KbOutMax=[]  KtOutMin=[]  KtOutMax=[]  IntegratorOutMin=[]  IntegratorOutMax=[]  FilterOutMin=[]  FilterOutMax=[]  SumI1OutMin=[]  SumI1OutMax=[]  SumI2OutMin=[]  SumI2OutMax=[]  SumI3OutMin=[]  SumI3OutMax=[]  SumI4OutMin=[]  SumI4OutMax=[]  SumDOutMin=[]  SumDOutMax=[]  DifferentiatorOutMin=[]  DifferentiatorOutMax=[]  FilterDiffOutCoefMin=[]  FilterDiffOutCoefMax=[]  ReciprocalOutMin=[]  ReciprocalOutMax=[]  SumDenOutMin=[]  SumDenOutMax=[]  SumNumOutMin=[]  SumNumOutMax=[]  DivideOutMin=[]  DivideOutMax=[]  UdiffTsProdOutMin=[]  UdiffTsProdOutMax=[]  NTsProdOutMin=[]  NTsProdOutMax=[]  UintegralTsProdOutMin=[]  UintegralTsProdOutMax=[]  UngainTsProdOutMin=[]  UngainTsProdOutMax=[]  IntegratorContinuousStateAttributes=''  IntegratorStateMustResolveToSignalObject=off  IntegratorRTWStateStorageClass=Auto  FilterContinuousStateAttributes=''  FilterStateMustResolveToSignalObject=off  FilterRTWStateStorageClass=Auto  ParallelPVariant=InternalParameters  IdealPVariant=Disabled  IVariant=InternalParameters  DVariant=InternalParameters  IntegratorVariant=Continuous  SatVariant=Disabled  AWVariant=Passthrough  PCopyVariant=Disabled  TRVariant=Disabled  FdbkBlocksVariant=Forward  IdealPFdbkVariant=Disabled  SatFdbkVariant=Disabled  DerivativeFilterVariant=ContFilter  NVariant=InternalParameters  NCopyVariant=Disabled  FilterICVariant=InternalICsFilter  IntegratorICVariant=InternalICs  ExternalResetVariant=Disabled  TRSumVariant=Passthrough  SumFdbkVariant=Disabled  SumVariant=Sum_PID  TsampFilterVariant=InternalTs  TsampNgainVariant=Passthrough  TsampIntegralVariant=Passthrough
  Rotation Matrix (R(fi)) : MATLAB Function  Commented=on  TreatAsAtomicUnit=on
  Scope : Scope
  Scope2 : Scope
  Selector : Selector  InputPortWidth=3  IndexOptions=Index vector (dialog)  Indices=[1 2]  OutputSizes=1
  Sum1 : Sum  Inputs=|+-
  Sum3 : Sum  Inputs=|+-
  Switch1 : Switch  Criteria=u2 ~= 0
  Switch4 : Switch  Criteria=u2 ~= 0
  Terminator : Terminator
  Terminator7 : Terminator
  Trajectory velocity generation1 : MATLAB Function  TreatAsAtomicUnit=on
  controller1 : MATLAB Function  Commented=on  TreatAsAtomicUnit=on
  es theta calculation : MATLAB Function  TreatAsAtomicUnit=on
  forward kinematic : MATLAB Function  TreatAsAtomicUnit=on
  invers Rotation Matrix (R(fi)) : MATLAB Function  Commented=on  TreatAsAtomicUnit=on
  invers kinematic : MATLAB Function  TreatAsAtomicUnit=on
  fi_dot1 : Outport
  robotPose1 : Outport  Port=2
  desiredVel1 : Outport  Port=3
  desiredPose1 : Outport  Port=4
  wires:
  invers kinematic/2(fi_L_dot) -> Mux1/2
  Constant3/1 -> Mux1/3
  Demux7/2 -> forward kinematic/3(fi_L_dot)
  Demux2/2 -> Terminator7/1
  w_measure1/1 -> Demux2/1
  t1/1 -> [t], Trajectory velocity generation1/1(t)
  Vmax1/1 -> Trajectory velocity generation1/3(Vmax)
  Constant4/1 -> Switch4/1
  Demux2/1 -> Demux7/1
  Demux7/1 -> forward kinematic/2(fi_R_dot)
  resetPose1/1 -> Integrator2/2, Integrator3/2
  angAccel1/1 -> Trajectory velocity generation1/6(angAccel)
  Switch1/1 -> Display5/1
  omegaMax1/1 -> Trajectory velocity generation1/5(omegaMax)
  Mux1/1 -> fi_dot1/1
  terminalPose1/1 -> Trajectory velocity generation1/7(terminalPose)
  departPose1/1 -> Trajectory velocity generation1/8(departPose)
  Trajectory velocity generation1/1(X_r_dot) -> desiredVel1/1, Integrator2/1
  Integrator2/1 -> Selector/1, desiredPose1/1, Demux5/1
  t_dep1/1 -> Trajectory velocity generation1/2(t_dep)
  Demux8/2 -> Switch4/3
  Constant2/1 -> Switch1/1
  Demux5/2 -> Switch1/3
  manual1/1 -> Switch4/2, Switch1/2
  accel1/1 -> Trajectory velocity generation1/4(accel)
  invers kinematic/1(fi_R_dot) -> Mux1/1
  Integrator3/1 -> Demux8/1, robotPose1/1
  Demux5/1 -> Terminator/1
  Demux8/1 -> Scope2/1, Sum3/2
  es theta calculation/1(es) -> PID Controller/1
  Sum1/1 -> PID Controller1/1
  PID Controller1/1 -> invers kinematic/2(w)
  PID Controller/1 -> invers kinematic/1(v)
  Selector/1 -> Scope/1, Sum3/1
  Sum3/1 -> Demux1/1
  Demux1/1 -> es theta calculation/1(dx)
  Demux1/2 -> es theta calculation/2(dy)
  Switch4/1 -> forward kinematic/1(fi), es theta calculation/3(fi), Sum1/2
  es theta calculation/2(fid) -> Sum1/1
  forward kinematic/1(X_R_dot) -> Integrator3/1

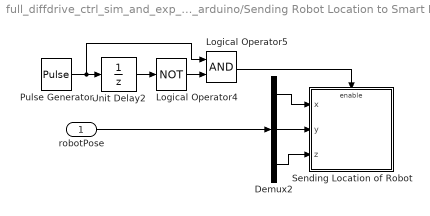
== system full_diffdrive_ctrl_sim_and_exp_with_arduino/Sending Robot Location to Smart Phone ==
  robotPose : Inport
  Demux2 : Demux  Outputs=3
  Logical Operator4 : Logic  Operator=NOT  AllPortsSameDT=off  OutDataTypeStr=boolean
  Logical Operator5 : Logic  AllPortsSameDT=off  OutDataTypeStr=boolean
  Pulse Generator : DiscretePulseGenerator  PulseType=Time based  Period=5  PulseWidth=50
  Sending Location of Robot : Subsystem
  Unit Delay2 : UnitDelay  SampleTime=-1  HasFrameUpgradeWarning=on
  wires:
  Demux2/3 -> Sending Location of Robot/3(z)
  Demux2/2 -> Sending Location of Robot/2(y)
  Demux2/1 -> Sending Location of Robot/1(x)
  Logical Operator5/1 -> Sending Location of Robot/Enable
  robotPose/1 -> Demux2/1
  Pulse Generator/1 -> Logical Operator5/1, Unit Delay2/1
  Unit Delay2/1 -> Logical Operator4/1
  Logical Operator4/1 -> Logical Operator5/2

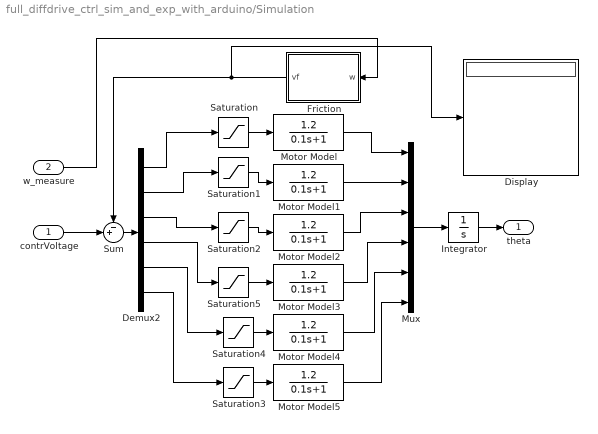
== system full_diffdrive_ctrl_sim_and_exp_with_arduino/Simulation ==
  contrVoltage : Inport
  w_measure : Inport  Port=2
  Demux2 : Demux  Outputs=6
  Display : Display
  Friction : MATLAB Function  TreatAsAtomicUnit=on
  Integrator : Integrator  InitialCondition=zeros(6,1)
  Motor Model{,1..5} (6 alike) : TransferFcn  Numerator=[1.2]  Denominator=[0.1 1]
  Mux : Mux  Inputs=6
  Saturation{,1..5} (6 alike) : Saturate  UpperLimit=19  LowerLimit=-19
  Sum : Sum  Inputs=-+|
  theta : Outport
  wires:
  contrVoltage/1 -> Sum/2
  Demux2/1 -> Saturation/1
  Motor Model2/1 -> Mux/3
  Motor Model3/1 -> Mux/4
  Motor Model4/1 -> Mux/5
  Motor Model5/1 -> Mux/6
  Demux2/2 -> Saturation1/1
  Demux2/3 -> Saturation2/1
  Demux2/4 -> Saturation5/1
  Demux2/5 -> Saturation4/1
  Demux2/6 -> Saturation3/1
  Mux/1 -> Integrator/1
  Friction/1(vf) -> Display/1, Sum/1
  Sum/1 -> Demux2/1
  w_measure/1 -> Friction/1(w)
  Integrator/1 -> theta/1
  Motor Model/1 -> Mux/1
  Motor Model1/1 -> Mux/2
  Saturation/1 -> Motor Model/1
  Saturation1/1 -> Motor Model1/1
  Saturation2/1 -> Motor Model2/1
  Saturation3/1 -> Motor Model5/1
  Saturation4/1 -> Motor Model4/1
  Saturation5/1 -> Motor Model3/1

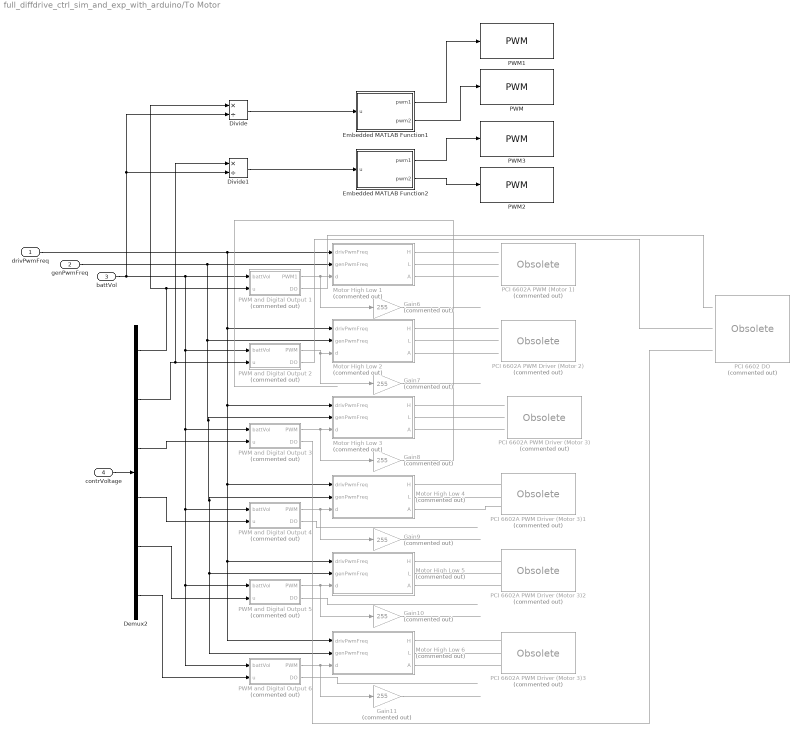
== system full_diffdrive_ctrl_sim_and_exp_with_arduino/To Motor ==
  drivPwmFreq : Inport
  genPwmFreq : Inport  Port=2
  battVol : Inport  Port=3
  contrVoltage : Inport  Port=4
  Demux2 : Demux  Outputs=6
  Divide : Product  Inputs=*/
  Divide1 : Product  Inputs=*/
  Embedded MATLAB Function1 : MATLAB Function  TreatAsAtomicUnit=on
  Embedded MATLAB Function2 : MATLAB Function  TreatAsAtomicUnit=on
  Gain{6..11} (6 alike) : Gain  Commented=on  Gain=255
  Motor High Low 1 : MATLAB Function  Commented=on  TreatAsAtomicUnit=on
  Motor High Low 2 : MATLAB Function  Commented=on  TreatAsAtomicUnit=on
  Motor High Low 3 : MATLAB Function  Commented=on  TreatAsAtomicUnit=on
  Motor High Low 4 : MATLAB Function  Commented=on  TreatAsAtomicUnit=on
  Motor High Low 5 : MATLAB Function  Commented=on  TreatAsAtomicUnit=on
  Motor High Low 6 : MATLAB Function  Commented=on  TreatAsAtomicUnit=on
  "PCI 6602 DO " : xpcobsoletelib/Obsolete  Commented=on
      settings: SourceProductBaseCode=XP
  PCI 6602A PWM (Motor 1) : xpcobsoletelib/Obsolete  Commented=on
      settings: SourceProductBaseCode=XP
  PCI 6602A PWM Driver (Motor 2) : xpcobsoletelib/Obsolete  Commented=on
      settings: SourceProductBaseCode=XP
  PCI 6602A PWM Driver (Motor 3){,1..3} (4 alike) : xpcobsoletelib/Obsolete  Commented=on
      settings: SourceProductBaseCode=XP
  PWM : arduinolib/PWM  pinNumber=6  frequencyType=Default  desiredFrequency=490.2  achievableFrequency=490.2
  PWM and Digital Output 1 : MATLAB Function  Commented=on  TreatAsAtomicUnit=on
  PWM and Digital Output 2 : MATLAB Function  Commented=on  TreatAsAtomicUnit=on
  PWM and Digital Output 3 : MATLAB Function  Commented=on  TreatAsAtomicUnit=on
  PWM and Digital Output 4 : MATLAB Function  Commented=on  TreatAsAtomicUnit=on
  PWM and Digital Output 5 : MATLAB Function  Commented=on  TreatAsAtomicUnit=on
  PWM and Digital Output 6 : MATLAB Function  Commented=on  TreatAsAtomicUnit=on
  PWM1 : arduinolib/PWM  pinNumber=7  frequencyType=Default  desiredFrequency=490.2  achievableFrequency=490.2
  PWM2 : arduinolib/PWM  pinNumber=4  frequencyType=Default  desiredFrequency=490.2  achievableFrequency=490.2
  PWM3 : arduinolib/PWM  pinNumber=5  frequencyType=Default  desiredFrequency=490.2  achievableFrequency=490.2
  wires:
  Motor High Low 6/2(L) -> ?
  PWM and Digital Output 6/1(PWM) -> Gain11/1, Motor High Low 6/3(d)
  drivPwmFreq/1 -> Motor High Low 6/1(drivPwmFreq), Motor High Low 5/1(drivPwmFreq), Motor High Low 4/1(drivPwmFreq), Motor High Low 3/1(drivPwmFreq), Motor High Low 2/1(drivPwmFreq), Motor High Low 1/1(drivPwmFreq)
  Gain11/1 -> ?
  genPwmFreq/1 -> Motor High Low 6/2(genPwmFreq), Motor High Low 5/2(genPwmFreq), Motor High Low 4/2(genPwmFreq), Motor High Low 3/2(genPwmFreq), Motor High Low 2/2(genPwmFreq), Motor High Low 1/2(genPwmFreq)
  Demux2/4 -> PWM and Digital Output 4/2(u)
  Demux2/5 -> PWM and Digital Output 5/2(u)
  PWM and Digital Output 4/1(PWM) -> Gain9/1, Motor High Low 4/3(d)
  Gain9/1 -> ?
  PWM and Digital Output 3/2(DO) -> ?
  battVol/1 -> Divide/2, Divide1/2, PWM and Digital Output 2/1(battVol), PWM and Digital Output 3/1(battVol), PWM and Digital Output 4/1(battVol), PWM and Digital Output 5/1(battVol), PWM and Digital Output 6/1(battVol), PWM and Digital Output 1/1(battVol)
  Demux2/3 -> PWM and Digital Output 3/2(u)
  Demux2/6 -> PWM and Digital Output 6/2(u)
  Motor High Low 5/1(H) -> ?
  contrVoltage/1 -> Demux2/1
  Motor High Low 5/3(A) -> ?
  PWM and Digital Output 3/1(PWM) -> Motor High Low 3/3(d), Gain8/1
  PWM and Digital Output 1/1(PWM1) -> Motor High Low 1/3(d), Gain6/1
  Motor High Low 6/3(A) -> ?
  Gain10/1 -> ?
  Motor High Low 2/2(L) -> ?
  Gain8/1 -> ?
  Motor High Low 2/3(A) -> ?
  PWM and Digital Output 5/1(PWM) -> Motor High Low 5/3(d), Gain10/1
  Motor High Low 4/1(H) -> ?
  PWM and Digital Output 2/1(PWM) -> Gain7/1, Motor High Low 2/3(d)
  Motor High Low 3/3(A) -> ?
  PWM and Digital Output 2/2(DO) -> ?
  Demux2/1 -> Divide/1, PWM and Digital Output 1/2(u)
  Gain7/1 -> ?
  Motor High Low 3/2(L) -> ?
  PWM and Digital Output 5/2(DO) -> ?
  PWM and Digital Output 4/2(DO) -> ?
  Motor High Low 4/2(L) -> ?
  PWM and Digital Output 6/2(DO) -> ?
  Motor High Low 3/1(H) -> ?
  Motor High Low 4/3(A) -> ?
  PWM and Digital Output 1/2(DO) -> ?
  Gain6/1 -> ?
  Motor High Low 5/2(L) -> ?
  Motor High Low 2/1(H) -> ?
  Motor High Low 6/1(H) -> ?
  Motor High Low 1/3(A) -> ?
  Motor High Low 1/2(L) -> ?
  Motor High Low 1/1(H) -> ?
  Divide1/1 -> Embedded MATLAB Function2/1(u)
  Divide/1 -> Embedded MATLAB Function1/1(u)
  Demux2/2 -> Divide1/1, PWM and Digital Output 2/2(u)
  Embedded MATLAB Function1/1(pwm1) -> PWM1/1
  Embedded MATLAB Function1/2(pwm2) -> PWM/1
  Embedded MATLAB Function2/1(pwm1) -> PWM3/1
  Embedded MATLAB Function2/2(pwm2) -> PWM2/1

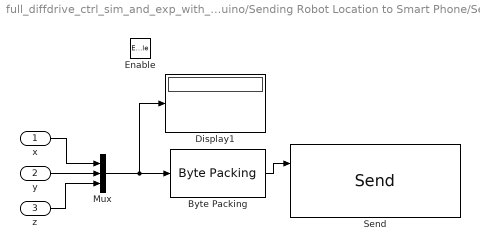
== system full_diffdrive_ctrl_sim_and_exp_with_arduino/Sending Robot Location to Smart Phone/Sending Location of Robot ==
  x : Inport
  y : Inport  Port=2
  z : Inport  Port=3
  Enable : EnablePort
  "Byte Packing " : xpcutilitieslib/Byte Packing   MaskPackedDataType=uint8  MaskUnpackedDataTypes={'double'}  MaskAlignment=1
  Display1 : Display
  Mux : Mux  Inputs=3
  "Send " : slrtlib/UDP/Send   localPort=-1  ipAddress=192.168.88.233  ipPort=2500  sampletime=-1
      settings: SourceProductBaseCode=XP
  wires:
  "Byte Packing "/1 -> "Send "/1
  Mux/1 -> Display1/1, "Byte Packing "/1
  y/1 -> Mux/2
  z/1 -> Mux/3
  x/1 -> Mux/1

== matlab function full_diffdrive_ctrl_sim_and_exp_with_arduino/To Motor/PWM and Digital Output 3 ==
  data: battVol input; u input; PWM output; DO output
function [PWM, DO]= fcn(battVol,u)   %PWM & D(Digital output) are the output and u is the input (Voltage=24V(because DC motor 24V)).
PWM = abs(u)/battVol;               % PWM equals to value of u (voltage value which was applied)
DO = (sign(u)+1)/2;          % (sign(u): included value of u and its sign)so we will get digital ouput between 0 and 1 (if u = 1 => D = 1 or if u = -1 => D =0)

== matlab function full_diffdrive_ctrl_sim_and_exp_with_arduino/To Motor/Motor High Low 4 ==
  data: drivPwmFreq input; genPwmFreq input; d input; H output; L output; A output
function [H,L,A]=fcn(drivPwmFreq,genPwmFreq,d)
%genPwmFreq = fm = 80e6;%refrence
%drivPwmFreq = f = 400;%desire
x = genPwmFreq/drivPwmFreq;
H = d*x;
L = (1-d)*x;
A = 1;

== matlab function full_diffdrive_ctrl_sim_and_exp_with_arduino/To Motor/PWM and Digital Output 4 ==
  data: battVol input; u input; PWM output; DO output
function [PWM, DO]= fcn(battVol,u)   %PWM & D(Digital output) are the output and u is the input (Voltage=24V(because DC motor 24V)).
PWM = abs(u)/battVol;               % PWM equals to value of u (voltage value which was applied)
DO = (sign(u)+1)/2;          % (sign(u): included value of u and its sign)so we will get digital ouput between 0 and 1 (if u = 1 => D = 1 or if u = -1 => D =0)

== matlab function full_diffdrive_ctrl_sim_and_exp_with_arduino/To Motor/Motor High Low 5 ==
  data: drivPwmFreq input; genPwmFreq input; d input; H output; L output; A output
function [H,L,A]=fcn(drivPwmFreq,genPwmFreq,d)
%genPwmFreq = fm = 80e6;%refrence
%drivPwmFreq = f = 400;%desire
x = genPwmFreq/drivPwmFreq;
H = d*x;
L = (1-d)*x;
A = 1;

== matlab function full_diffdrive_ctrl_sim_and_exp_with_arduino/To Motor/PWM and Digital Output 1 ==
  data: battVol input; u input; PWM1 output; DO output
function [PWM1, DO]= fcn(battVol,u)   %PWM & D(Digital output) are the output and u is the input (Voltage=24V(because DC motor 24V)).
PWM = abs(u)/battVol;               % PWM equals to value of u (voltage value which was applied)
DO = (sign(u)+1)/2;          % (sign(u): included value of u and its sign)so we will get digital ouput between 0 and 1 (if u = 1 => D = 1 or if u = -1 => D =0)
